simulink model "sprawko2_sim"  (R2025b)
settings: Solver=VariableStepAuto  StartTime=0.0  StopTime=500  MaxStep=1  RelTol=1e-3
values from neighbouring files (symbols this model uses):
  k = delta_x / delta_u    [skrypt3.m]    (also in skrypt4.m)
  przy_kz = 0    [skrypt2.m]    (also in skrypt3.m = 1; skrypt4.m = 1)
  step_time = 400    [skrypt2.m]    (also in skrypt3.m = 10; skrypt4.m = 100)
  T = 247    [skrypt3.m]    (also in skrypt4.m)
  t_0 = 13    [skrypt3.m]    (also in skrypt4.m)
  Tw2c = ((A + Ks1 + K0)*Ks2*Tzew0 + K0*(A*Tkz0 + Ks1*Tzew0)) / ((A + Ks1 + K0)*(K0 + Ks2) - K0^2)    [skrypt2.m]    (also in skrypt3.m = 15; skrypt4.m = 15)
settings Model: Creator=mikol  LastModifiedBy=mikol

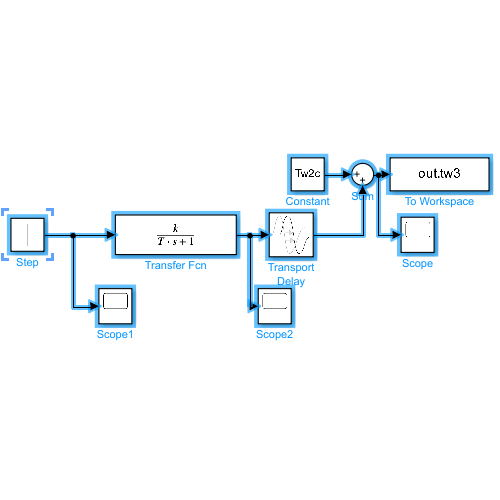
[thumbnail: Simulink's stored preview of the top-level diagram]
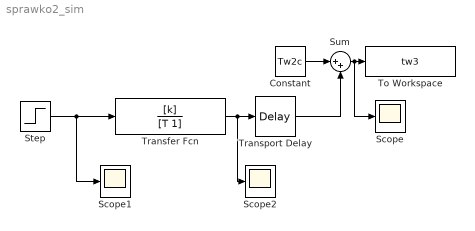
== system sprawko2_sim ==
  Constant : Constant  Value=Tw2c
  Scope : Scope
      settings: ActiveDisplayYMinimum=14.238082536293582  ActiveDisplayYMaximum=33.083673858522125
  Scope1 : Scope
      settings: ActiveDisplayYMinimum=-1  ActiveDisplayYMaximum=1
  Scope2 : Scope
      settings: ActiveDisplayYMinimum=-1  ActiveDisplayYMaximum=1  DataLoggingVariableName=ScopeData2
  Step : Step  Time=step_time  After=przy_kz  SampleTime=0
  Sum : Sum  Inputs=|++
  To Workspace : ToWorkspace  VariableName=tw3  SaveFormat=Timeseries  SampleTime=-1
  Transfer Fcn : TransferFcn  Numerator=[k]  Denominator=[T 1]
  Transport Delay : TransportDelay  DelayTime=t_0
  wires:
  Step/1 -> Transfer Fcn/1, Scope1/1
  Constant/1 -> Sum/1
  Sum/1 -> Scope/1, To Workspace/1
  Transfer Fcn/1 -> Scope2/1, Transport Delay/1
  Transport Delay/1 -> Sum/2
